simulink model "Matlab_Motor_DC_Excitation"  (R2016a)
settings: Solver=VariableStepAuto  StartTime=0.0  StopTime=5  RelTol=1e-3
libraries: powerlib x12
settings Model: Creator=Douglas  LastModifiedBy=Douglas

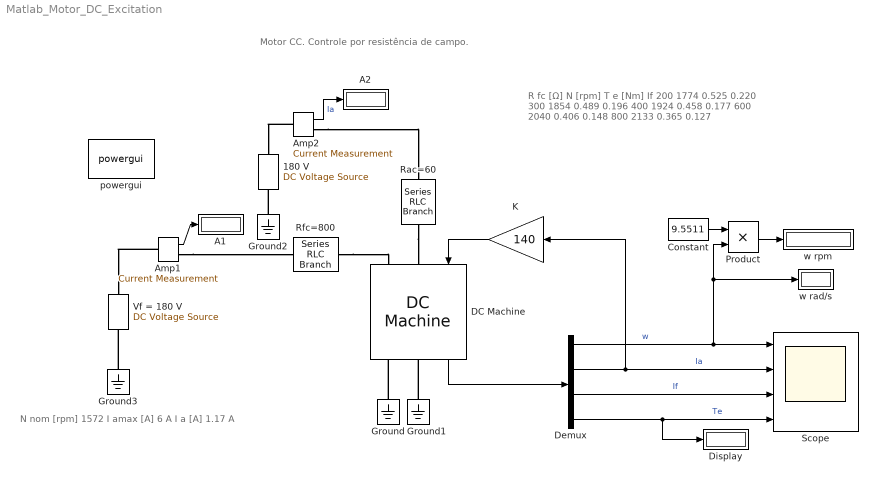
== system Matlab_Motor_DC_Excitation ==
  note: R fc [Ω]
      | N [rpm]
      | T e [Nm]
      | If
      |
      | 200
      | 1774
      | 0.525
      | 0.220
      |
      | 300
      | 1854
      | 0.489
      | 0.196
      |
      | 400
      | 1924
      | 0.458
      | 0.177
      |
      | 600
      | 2040
      | 0.406
      | 0.148
      |
      | 800
      | 2133
      | 0.365
      | 0.127
  note: N nom [rpm]
      | 1572
      |
      | I amax [A]
      | 6 A
      |
      | I a [A]
      | 1.17 A
  note: Motor CC. Controle por resistência de campo.
  180 V : powerlib/Electrical Sources/DC Voltage Source  Amplitude=185  Measurements=None
  A1 : Display
  A2 : Display
  Amp1 : powerlib/Measurements/Current Measurement  PhasorSimulation=off  OutputType=Complex  PSBequivalent=0
  Amp2 : powerlib/Measurements/Current Measurement  PhasorSimulation=off  OutputType=Complex  PSBequivalent=0
  Constant : Constant  Value=9.5511
  DC Machine : powerlib/Machines/DC Machine  PresetModel=No  MechanicalLoad=Speed w  FieldType=Wound  ShowDetailedParameters=on  MeasurementBus=off  RLa="[ 24  0.0]"  RLf="[ 618  0.05]"  Laf=1.8  MachineConstant=Torque constant (N.m/A)  Ke=1.8  Kt=1.8  J=1  Bm=0  Tf=0  w0=1  Ifinit=0.3  TsPowergui=0  TsBlock=-1
  Demux : Demux
  Display : Display
  Ground{,1..3} (4 alike) : powerlib/Elements/Ground  LConnTagsString=a
  K : Gain  Gain=140
  Product : Product
  Rac=60 : powerlib/Elements/Series RLC Branch  LConnTagsString=__new0  RConnTagsString=__new0  BranchType=R  Resistance=60  Inductance=1e-3  SetiL0=off  InitialCurrent=0  Capacitance=1e-6  Setx0=off  InitialVoltage=0  Measurements=None
  Rfc=800 : powerlib/Elements/Series RLC Branch  LConnTagsString=__new0  RConnTagsString=__new0  BranchType=R  Resistance=800  Inductance=1e-3  SetiL0=off  InitialCurrent=0  Capacitance=1e-6  Setx0=off  InitialVoltage=0  Measurements=None
  Scope : Scope  NumInputPorts=4
  Vf = 180 V : powerlib/Electrical Sources/DC Voltage Source  Amplitude=180  Measurements=None
  powergui : powerlib/powergui  Priority=1  SimulationMode=Discrete  SolverType=Tustin/Backward Euler (TBE)  SampleTime=50e-6  frequency=60  SPID=off  DisableSnubberDevices=off  DisableRonSwitches=off  DisableVfSwitches=off  SwTol=0  DisplayEquations=off  Interpol=off  ExternalGateDelay=off  methode=off  Ts=10  FunctionMessages=off  echomessages=off  HookPort=off  EnableUseOfTLC=off  x0status=blocks  frequencyindice=0  Pbase=100e6  ErrMax=1e-4  Iterations=50  UnitsV=kV  UnitsW=MW  buscounter=0  RestoreLinks=warning  ResistiveCurrentMeasurement=off  Frange=[0:2:500]  Ylog=off  Xlog=on  ShowGrid=off  save=off  variable=ZData  structure=0  ZoomFFT=off  StartTime=0.0  cycles=1  DisplayStyle=1  fundamental=60  FreqAxis=off  MaxFrequency=1000  frequencyindicesteady=1  RmsSteady=1  display=off
  w rad/s : Display
  w rpm : Display
  wires:
  DC Machine/1 -> Demux/1
  Demux/3 -> Scope/3  "If"
  Demux/4 -> Scope/4, Display/1  "Te"
  Demux/1 -> w rad/s/1, Product/2, Scope/1  "w"
  Demux/2 -> K/1, Scope/2  "Ia"
  Constant/1 -> Product/1
  Product/1 -> w rpm/1
  Amp1/1 -> A1/1
  Amp2/1 -> A2/1  "Ia"
  K/1 -> DC Machine/1
  connections:
  Ground/LConn1 -- DC Machine/RConn2
  Ground1/LConn1 -- DC Machine/RConn1
  Ground2/LConn1 -- 180 V/LConn1
  Rac=60/RConn1 -- DC Machine/LConn1
  Ground3/LConn1 -- Vf = 180 V/LConn1
  Rfc=800/LConn1 -- DC Machine/LConn2
  Amp1/RConn1 -- Rfc=800/RConn1
  Amp1/LConn1 -- Vf = 180 V/RConn1
  Amp2/LConn1 -- 180 V/RConn1
  Amp2/RConn1 -- Rac=60/LConn1
